simulink model "testFrame_CalcSpeednDir"  (R2020b)
settings: Solver=FixedStepDiscrete  StartTime=0.0  StopTime=10.0  FixedStep=200e-6  RelTol=1e-3
settings Model: PacingRate=100  Creator=unix  LastModifiedBy=unix

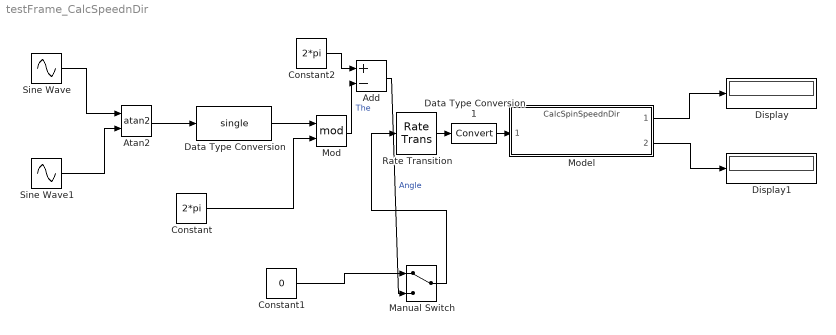
== system testFrame_CalcSpeednDir ==
  Add : Sum  Inputs=+-
  Atan2 : Trigonometry  Operator=atan2
  Constant : Constant  Value=2*pi  OutDataTypeStr=single
  Constant1 : Constant  Value=0  OutDataTypeStr=single
  Constant2 : Constant  Value=2*pi  OutDataTypeStr=Inherit: Inherit via back propagation
  Data Type Conversion : DataTypeConversion  OutDataTypeStr=single
  Data Type Conversion1 : DataTypeConversion
  Display : Display
  Display1 : Display
  Manual Switch : ManualSwitch
  Mod : Math  Operator=mod  SaturateOnIntegerOverflow=on
  Model : ModelReference  ModelNameDialog=CalcSpinSpeednDir.slx  ModelReferenceVersion=3.23
  Rate Transition : RateTransition
  Sine Wave : Sin  Frequency=100  SampleTime=0
  Sine Wave1 : Sin  Frequency=100  Phase=pi/2  SampleTime=0
  wires:
  Sine Wave/1 -> Atan2/1
  Sine Wave1/1 -> Atan2/2
  Atan2/1 -> Data Type Conversion/1
  Data Type Conversion/1 -> Mod/1
  Constant/1 -> Mod/2
  Model/1 -> Display/1
  Model/2 -> Display1/1
  Constant2/1 -> Add/1
  Mod/1 -> Add/2  "The"
  Add/1 -> Manual Switch/2  "Angle"
  Constant1/1 -> Manual Switch/1
  Manual Switch/1 -> Rate Transition/1
  Rate Transition/1 -> Data Type Conversion1/1
  Data Type Conversion1/1 -> Model/1
